simulink model "sampleModel1683_3_sub_sub"  (R2023a)
settings: Solver=VariableStepAuto  StartTime=0.0  StopTime=10.0  RelTol=1e-3
libraries: hdlsllib x2
settings Model: Creator=user1  LastModifiedBy=user1
settings OptimizationCC: BlockReduction=off  ConditionallyExecuteInputs=off

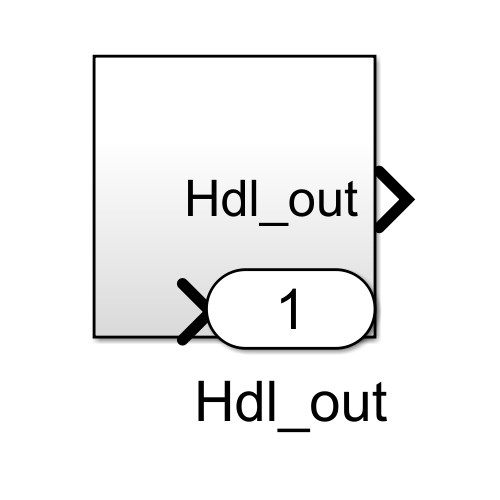
[thumbnail: Simulink's stored preview of the top-level diagram]
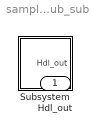
== system sampleModel1683_3_sub_sub ==
  Subsystem : Subsystem
  Hdl_out : Outport  OutDataTypeStr=uint8

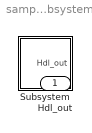
== system sampleModel1683_3_sub_sub/Subsystem ==
  Subsystem : Subsystem
  Hdl_out : Outport  OutDataTypeStr=uint8

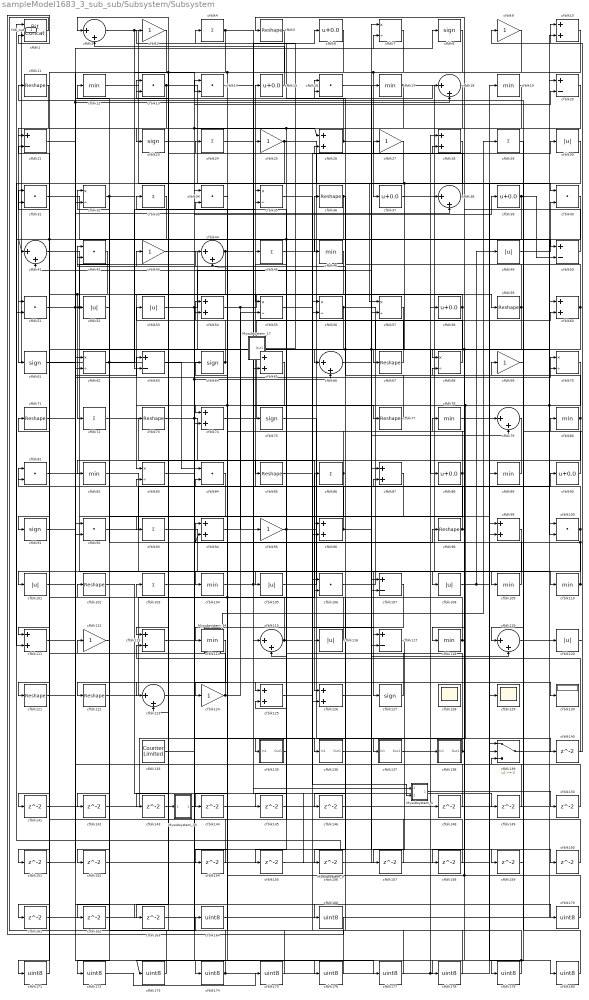
== system sampleModel1683_3_sub_sub/Subsystem/Subsystem ==
  Mysubsystem_17 : Subsystem  TreatAsAtomicUnit=on  RTWFcnName=Mysubsystem_17
      settings: RTWFcnNameOpts=User specified  RTWFileNameOpts=Use function name
  Mysubsystem_33 : Subsystem  TreatAsAtomicUnit=on  RTWFcnName=Mysubsystem_33
      settings: RTWFcnNameOpts=User specified  RTWFileNameOpts=Use function name
  Mysubsystem_34 : Subsystem  TreatAsAtomicUnit=on  RTWFcnName=Mysubsystem_34
      settings: RTWFcnNameOpts=User specified  RTWFileNameOpts=Use function name
  Mysubsystem_4 : Subsystem  TreatAsAtomicUnit=on  RTWFcnName=Mysubsystem_4
      settings: RTWFcnNameOpts=User specified  RTWFileNameOpts=Use function name
  Mysubsystem_9 : Subsystem  TreatAsAtomicUnit=on  RTWFcnName=Mysubsystem_9
      settings: RTWFcnNameOpts=User specified  RTWFileNameOpts=Use function name
  cfblk1 : hdlsllib/Logic and Bit Operations/Bit Concat  numInputs=2
  cfblk{10,26,28,54,60,65,74,87,94,96,99,111,113,125..126} (15 alike) : Sum  OutDataTypeStr=uint8
  cfblk{13..14,16,31,34,40,42,51,81,84,92,100,106} (13 alike) : DotProduct  OutDataTypeStr=uint8
  cfblk{30,49,52..53,101,105,108,116,120} (9 alike) : Abs  OutDataTypeStr=uint8  SaturateOnIntegerOverflow=off
  cfblk{5,11,36,59,67,71,73,77,85,98,102,121..122} (13 alike) : Reshape
  cfblk{4,24,29,33,45,72,86,93,103} (9 alike) : Sum  Inputs=+  OutDataTypeStr=uint8
  cfblk{12,17,19,46,78,80,82,89,104,109..110,114,118} (13 alike) : MinMax  OutDataTypeStr=uint8
  cfblk{20..21,50,63,107,117} (6 alike) : Sum  Inputs=+-  OutDataTypeStr=uint8
  cfblk{3,9,25,27,43,69,95,112,124} (9 alike) : Gain  OutDataTypeStr=uint8
  cfblk{2,18,38,41,44,66,79,115,119,123} (10 alike) : Sum  Inputs=|++  OutDataTypeStr=uint8
  cfblk{8,23,61,64,75,91,127} (7 alike) : Signum
  cfblk128 : Scope
      settings: Floating=on
  cfblk129 : Scope
  cfblk130 : Display
  cfblk133 : hdlsllib/Sources/Counter Limited  uplimit=7  tsamp=-1
  cfblk135 : Subsystem
      settings: LibrarySourceBlock=|
      | hdlsllib/Ports &
      | Subsystems/Subsystem
  cfblk136 : Subsystem
      settings: LibrarySourceBlock=|
      | hdlsllib/Ports &
      | Subsystems/Subsystem
  cfblk137 : Subsystem
      settings: LibrarySourceBlock=|
      | hdlsllib/Ports &
      | Subsystems/Subsystem
  cfblk138 : Subsystem
      settings: LibrarySourceBlock=|
      | hdlsllib/Ports &
      | Subsystems/Subsystem
  cfblk139 : Switch  OutDataTypeStr=uint8  SaturateOnIntegerOverflow=off  InputSameDT=off
  cfblk{140..146,148..152,154..163} (22 alike) : Delay  SampleTime=1
  cfblk{6,15,37,39,58,88,90} (7 alike) : Bias  Bias=0.0  SaturateOnIntegerOverflow=off
  cfblk{164,166,170..180} (13 alike) : DataTypeConversion  OutDataTypeStr=uint8  SaturateOnIntegerOverflow=off  RndMeth=Floor
  cfblk{7,32,35,55..57,62,68,70,83} (10 alike) : Product  Inputs=*/  OutDataTypeStr=uint8  RndMeth=Zero  SaturateOnIntegerOverflow=on
  Hdl_out : Outport  OutDataTypeStr=uint8
  wires:
  Mysubsystem_34/1(Out1) -> cfblk29/1
  Mysubsystem_33/1(Out1) -> cfblk87/1
  Mysubsystem_17/1(Out1) -> cfblk4/1
  Mysubsystem_9/1(Out1) -> cfblk1/1
  cfblk102/1 -> Mysubsystem_9/1(In1)
  Mysubsystem_4/1(Out1) -> cfblk150/1
  cfblk24/1 -> Mysubsystem_4/1(In1)
  cfblk180/1 -> cfblk69/1
  cfblk78/1 -> cfblk180/1
  cfblk179/1 -> cfblk173/1, cfblk106/2
  cfblk178/1 -> cfblk103/1
  cfblk79/1 -> cfblk178/1
  cfblk177/1 -> cfblk106/1
  cfblk103/1 -> cfblk177/1
  cfblk176/1 -> cfblk34/2
  cfblk175/1 -> cfblk34/1
  cfblk172/1 -> cfblk175/1
  cfblk174/1 -> cfblk148/1, cfblk19/1, cfblk102/1
  cfblk173/1 -> cfblk112/1
  cfblk112/1 -> cfblk172/1
  cfblk171/1 -> cfblk71/1
  cfblk33/1 -> cfblk171/1
  cfblk170/1 -> cfblk68/2, cfblk84/2
  cfblk166/1 -> cfblk1/2
  cfblk162/1 -> cfblk166/1
  cfblk164/1 -> cfblk58/1
  cfblk1/1 -> cfblk164/1
  cfblk163/1 -> cfblk20/1
  cfblk46/1 -> cfblk163/1
  cfblk161/1 -> cfblk10/2
  cfblk160/1 -> cfblk28/2
  cfblk159/1 -> cfblk139/3
  cfblk158/1 -> cfblk125/2
  cfblk157/1 -> cfblk81/2
  cfblk117/1 -> cfblk157/1
  cfblk156/1 -> cfblk139/2
  cfblk155/1 -> cfblk57/2
  cfblk154/1 -> cfblk83/2
  cfblk152/1 -> cfblk79/1
  cfblk84/1 -> cfblk152/1
  cfblk151/1 -> cfblk32/2
  cfblk150/1 -> cfblk92/1
  cfblk149/1 -> cfblk62/1
  cfblk94/1 -> cfblk149/1
  cfblk148/1 -> cfblk13/2
  cfblk146/1 -> cfblk107/1
  cfblk145/1 -> cfblk56/1
  cfblk144/1 -> cfblk54/2
  cfblk7/1 -> cfblk144/1
  cfblk143/1 -> cfblk99/1
  cfblk18/1 -> cfblk143/1
  cfblk142/1 -> cfblk74/2
  cfblk114/1 -> cfblk142/1
  cfblk141/1 -> cfblk60/1
  cfblk140/1 -> cfblk113/2
  cfblk126/1 -> cfblk140/1
  cfblk107/1 -> cfblk124/1
  cfblk66/1 -> cfblk7/1
  cfblk58/1 -> cfblk92/2, cfblk96/1, cfblk52/1
  cfblk62/1 -> cfblk32/1, cfblk35/2
  cfblk88/1 -> cfblk35/1, cfblk156/1
  cfblk91/1 -> cfblk8/1
  cfblk40/1 -> cfblk115/2
  cfblk136/1(Out1) -> cfblk119/2
  cfblk89/1 -> cfblk85/1
  cfblk101/1 -> cfblk18/2, cfblk7/2
  cfblk16/1 -> cfblk79/2
  cfblk10/1 -> cfblk73/1
  cfblk31/1 -> cfblk46/1
  cfblk113/1 -> cfblk136/1(In1)
  cfblk35/1 -> cfblk117/1
  cfblk123/1 -> cfblk14/1
  cfblk55/1 -> cfblk70/2
  cfblk104/1 -> cfblk130/1, cfblk6/1
  cfblk125/1 -> cfblk87/2
  cfblk92/1 -> cfblk28/1
  cfblk21/1 -> cfblk18/1
  cfblk64/1 -> cfblk54/1, Hdl_out/1
  cfblk4/1 -> cfblk111/1, cfblk77/1
  cfblk115/1 -> Mysubsystem_4/2(In2), cfblk94/1, cfblk21/2
  cfblk51/1 -> cfblk39/1, cfblk88/1, cfblk176/1
  cfblk23/1 -> cfblk26/1, cfblk16/1
  cfblk100/1 -> cfblk94/2, cfblk121/1, cfblk42/2
  cfblk61/1 -> cfblk38/2
  cfblk87/1 -> cfblk116/1
  cfblk96/1 -> cfblk110/1, cfblk31/1
  cfblk124/1 -> cfblk81/1, cfblk55/2
  cfblk3/1 -> cfblk101/1, cfblk41/1
  cfblk93/1 -> cfblk127/1
  cfblk53/1 -> cfblk66/2, cfblk160/1, cfblk17/1
  cfblk9/1 -> cfblk44/2, cfblk123/2
  cfblk110/1 -> cfblk80/1, cfblk12/1
  cfblk106/1 -> cfblk38/1
  cfblk15/1 -> cfblk2/2
  cfblk111/1 -> cfblk70/1
  cfblk28/1 -> cfblk113/1
  cfblk5/1 -> cfblk62/2
  cfblk6/1 -> cfblk23/1, cfblk21/1
  cfblk135/1(Out1) -> cfblk45/1
  cfblk59/1 -> cfblk114/1, cfblk16/2
  cfblk65/1 -> cfblk104/1
  cfblk67/1 -> cfblk25/1
  cfblk25/1 -> cfblk51/2, cfblk117/2
  cfblk80/1 -> cfblk82/1, cfblk41/2
  cfblk39/1 -> cfblk111/2, cfblk155/1, cfblk50/2
  cfblk14/1 -> cfblk66/1
  cfblk81/1 -> cfblk99/2
  cfblk83/1 -> cfblk125/1
  cfblk34/1 -> cfblk174/1
  cfblk120/1 -> cfblk10/1
  cfblk32/1 -> cfblk56/2, cfblk162/1
  cfblk29/1 -> cfblk119/1
  cfblk108/1 -> cfblk89/1, cfblk49/1
  cfblk85/1 -> cfblk30/1
  cfblk37/1 -> cfblk100/1
  cfblk50/1 -> cfblk24/1
  cfblk49/1 -> cfblk40/2
  cfblk133/1 -> cfblk98/1
  cfblk20/1 -> cfblk74/1
  cfblk121/1 -> cfblk63/1
  cfblk13/1 -> cfblk139/1, cfblk161/1
  cfblk86/1 -> cfblk44/1, cfblk93/1
  cfblk19/1 -> cfblk91/1, cfblk55/1
  cfblk30/1 -> cfblk135/1(In1), cfblk67/1
  cfblk56/1 -> cfblk68/1, cfblk65/1
  cfblk119/1 -> cfblk120/1
  cfblk43/1 -> cfblk126/2
  cfblk54/1 -> cfblk59/1, cfblk95/1
  cfblk38/1 -> cfblk3/1
  cfblk60/1 -> cfblk118/1, cfblk96/2, cfblk26/2
  cfblk45/1 -> cfblk36/1
  cfblk122/1 -> cfblk86/1
  cfblk27/1 -> cfblk51/1
  cfblk90/1 -> cfblk11/1
  cfblk68/1 -> cfblk13/1
  cfblk69/1 -> cfblk179/1
  cfblk137/1(Out1) -> cfblk138/1(In1)
  cfblk12/1 -> cfblk40/1
  cfblk139/1 -> cfblk9/1
  cfblk73/1 -> cfblk126/1, cfblk20/2
  cfblk72/1 -> cfblk115/1
  cfblk42/1 -> cfblk72/1, cfblk151/1
  cfblk109/1 -> cfblk64/1
  cfblk26/1 -> cfblk2/1, cfblk159/1
  cfblk82/1 -> cfblk105/1
  cfblk52/1 -> cfblk122/1
  cfblk74/1 -> cfblk60/2
  cfblk138/1(Out1) -> cfblk43/1, cfblk158/1
  cfblk95/1 -> cfblk90/1, cfblk75/1
  cfblk77/1 -> cfblk42/1
  cfblk11/1 -> cfblk61/1
  cfblk71/1 -> cfblk170/1
  cfblk17/1 -> cfblk129/1, cfblk65/2
  cfblk98/1 -> cfblk15/1, cfblk78/1
  cfblk75/1 -> cfblk137/1(In1)
  cfblk116/1 -> cfblk53/1
  cfblk57/1 -> cfblk107/2, cfblk141/1
  cfblk44/1 -> cfblk83/1, cfblk50/1
  cfblk41/1 -> cfblk108/1
  cfblk36/1 -> cfblk145/1, cfblk146/1
  cfblk70/1 -> Mysubsystem_33/1(In1), cfblk123/1, cfblk154/1, cfblk100/2
  cfblk99/1 -> cfblk109/1
  cfblk63/1 -> cfblk84/1
  cfblk105/1 -> cfblk27/1
  cfblk118/1 -> cfblk5/1, cfblk31/2
  cfblk2/1 -> cfblk57/1, cfblk14/2
  cfblk8/1 -> cfblk37/1, cfblk63/2
  cfblk127/1 -> cfblk33/1

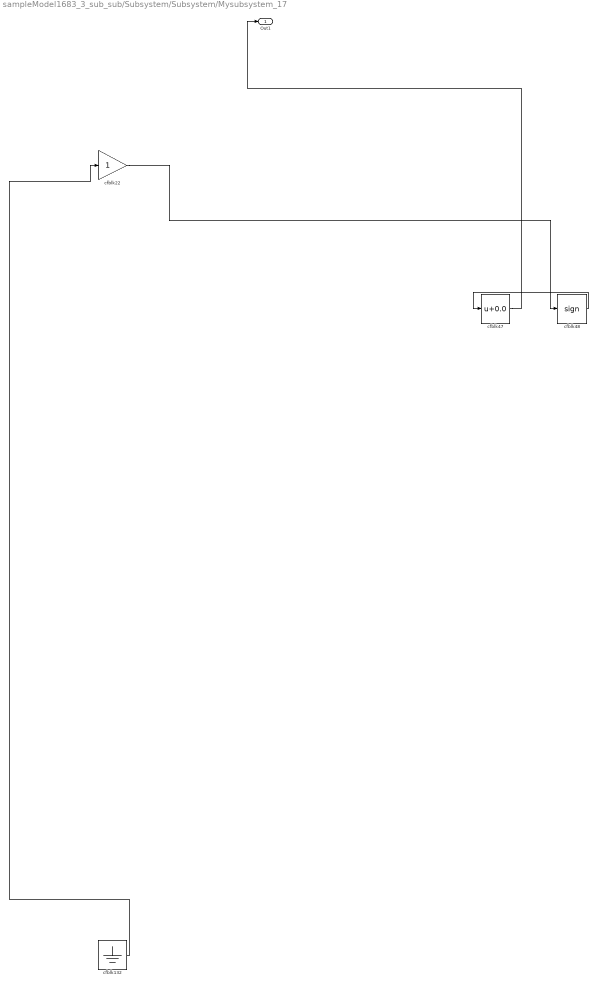
== system sampleModel1683_3_sub_sub/Subsystem/Subsystem/Mysubsystem_17 ==
  cfblk132 : Ground
  cfblk22 : Gain
  cfblk47 : Bias  Bias=0.0  SaturateOnIntegerOverflow=off
  cfblk48 : Signum
  Out1 : Outport
  wires:
  cfblk22/1 -> cfblk48/1
  cfblk47/1 -> Out1/1
  cfblk48/1 -> cfblk47/1
  cfblk132/1 -> cfblk22/1

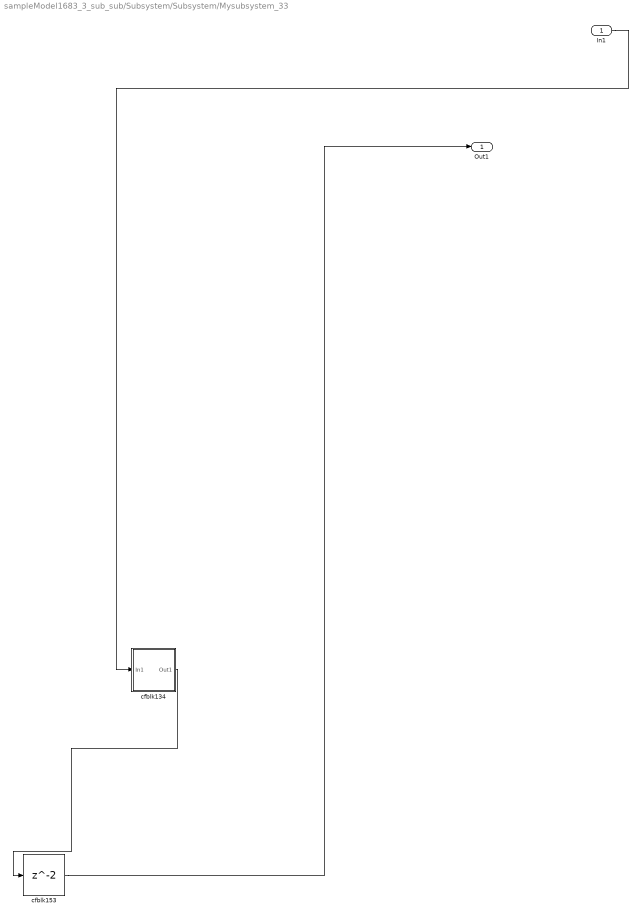
== system sampleModel1683_3_sub_sub/Subsystem/Subsystem/Mysubsystem_33 ==
  In1 : Inport
  cfblk134 : Subsystem
      settings: LibrarySourceBlock=|
      | hdlsllib/Ports &
      | Subsystems/Subsystem
  cfblk153 : Delay  SampleTime=1
  Out1 : Outport
  wires:
  cfblk134/1(Out1) -> cfblk153/1
  In1/1 -> cfblk134/1(In1)
  cfblk153/1 -> Out1/1

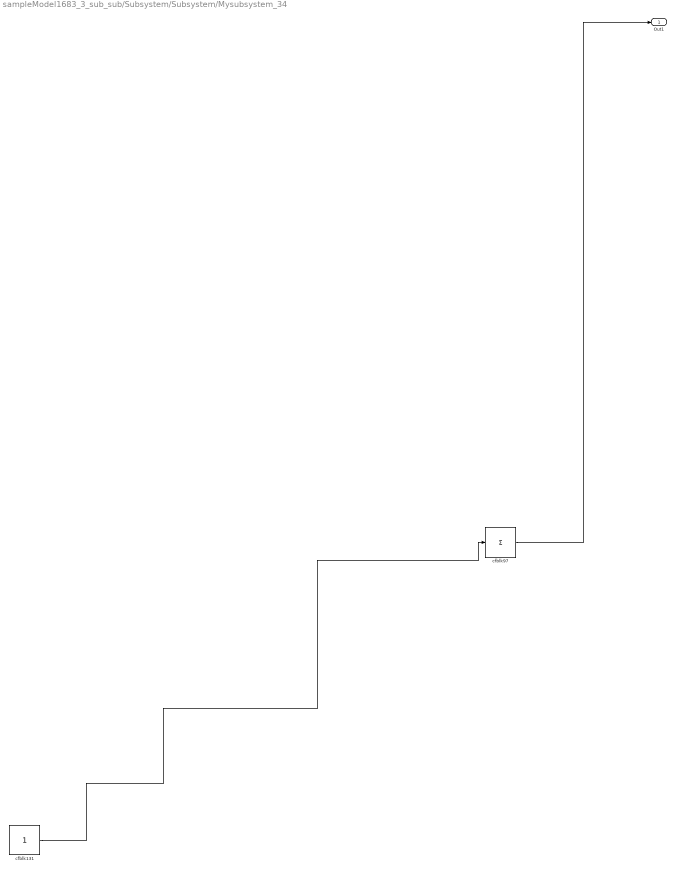
== system sampleModel1683_3_sub_sub/Subsystem/Subsystem/Mysubsystem_34 ==
  cfblk131 : Constant  SampleTime=-1
  cfblk97 : Sum  Inputs=+
  Out1 : Outport
  wires:
  cfblk97/1 -> Out1/1
  cfblk131/1 -> cfblk97/1

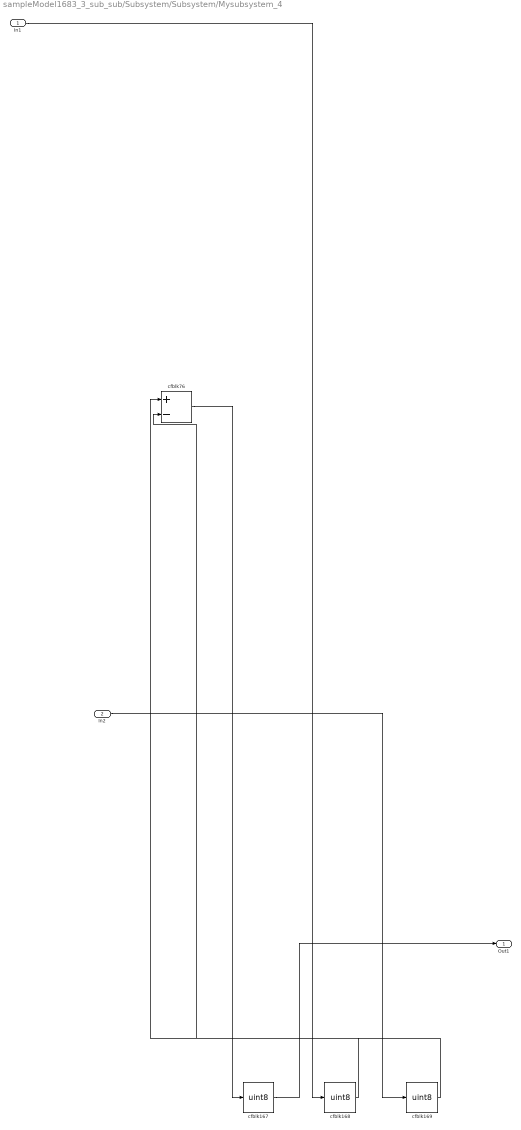
== system sampleModel1683_3_sub_sub/Subsystem/Subsystem/Mysubsystem_4 ==
  In1 : Inport
  In2 : Inport  Port=2
  cfblk167 : DataTypeConversion  OutDataTypeStr=uint8  SaturateOnIntegerOverflow=off  RndMeth=Floor
  cfblk168 : DataTypeConversion  OutDataTypeStr=uint8  SaturateOnIntegerOverflow=off  RndMeth=Floor
  cfblk169 : DataTypeConversion  OutDataTypeStr=uint8  SaturateOnIntegerOverflow=off  RndMeth=Floor
  cfblk76 : Sum  Inputs=+-
  Out1 : Outport
  wires:
  cfblk76/1 -> cfblk167/1
  cfblk168/1 -> cfblk76/1
  cfblk169/1 -> cfblk76/2
  cfblk167/1 -> Out1/1
  In2/1 -> cfblk169/1
  In1/1 -> cfblk168/1

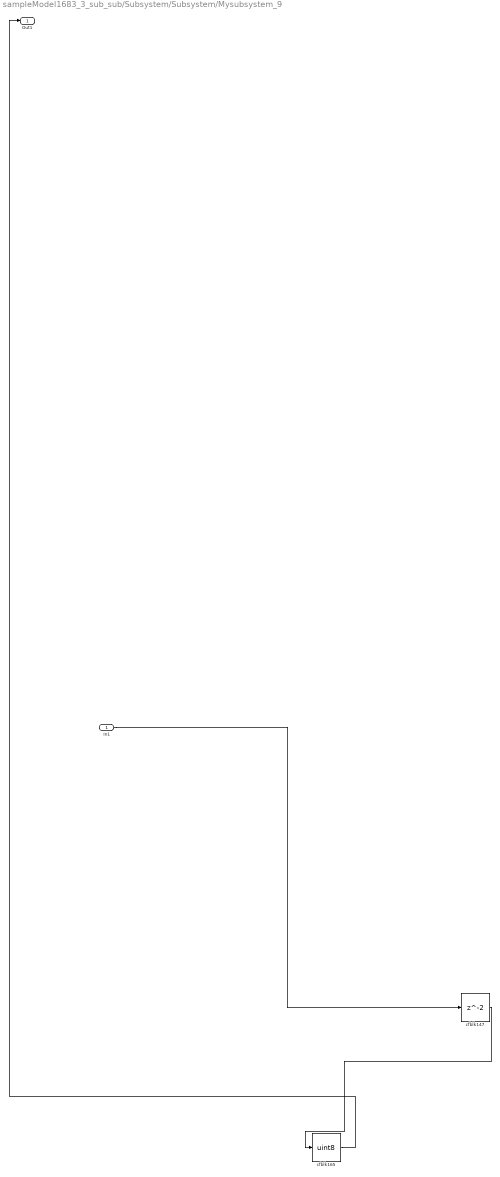
== system sampleModel1683_3_sub_sub/Subsystem/Subsystem/Mysubsystem_9 ==
  In1 : Inport
  cfblk147 : Delay  SampleTime=1
  cfblk165 : DataTypeConversion  OutDataTypeStr=uint8  SaturateOnIntegerOverflow=off  RndMeth=Floor
  Out1 : Outport
  wires:
  In1/1 -> cfblk147/1
  cfblk147/1 -> cfblk165/1
  cfblk165/1 -> Out1/1

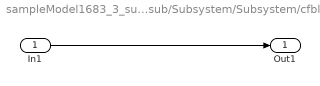
== system sampleModel1683_3_sub_sub/Subsystem/Subsystem/cfblk135 ==
  In1 : Inport
  Out1 : Outport
  wires:
  In1/1 -> Out1/1

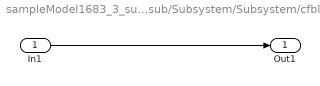
== system sampleModel1683_3_sub_sub/Subsystem/Subsystem/cfblk136 ==
  In1 : Inport
  Out1 : Outport
  wires:
  In1/1 -> Out1/1

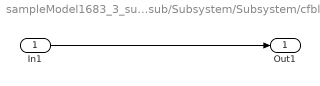
== system sampleModel1683_3_sub_sub/Subsystem/Subsystem/cfblk137 ==
  In1 : Inport
  Out1 : Outport
  wires:
  In1/1 -> Out1/1

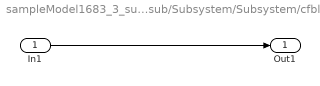
== system sampleModel1683_3_sub_sub/Subsystem/Subsystem/cfblk138 ==
  In1 : Inport
  Out1 : Outport
  wires:
  In1/1 -> Out1/1

== system sampleModel1683_3_sub_sub/Subsystem/Subsystem/Mysubsystem_33/cfblk134 ==
  In1 : Inport
  Out1 : Outport
  wires:
  In1/1 -> Out1/1
